simulink library "EnergyLimiterBtc"  (R2022b)
settings: Solver=VariableStepAuto  StartTime=0.0  StopTime=10.0  RelTol=1e-3
undefined symbols (not defined in the file or in its folder): magnitude
libraries: StateVar x5, AudioStats x1, FeaturePath x1, HandyTextFile x1, RTC x1
settings Model: Creator=kl13806  LastModifiedBy=kl13806
settings SolverCC: AlgebraicLoopSolver=TrustRegion
settings DebuggingCC: UnconnectedInputMsg=warning  UnconnectedOutputMsg=warning  UnconnectedLineMsg=warning  SFMachineParentedDataDiag=warning
settings ModelReferenceCC: EnableRefExpFcnMdlSchedulingChecks=on
settings RTWCC: DLArmComputeVersion=19.05

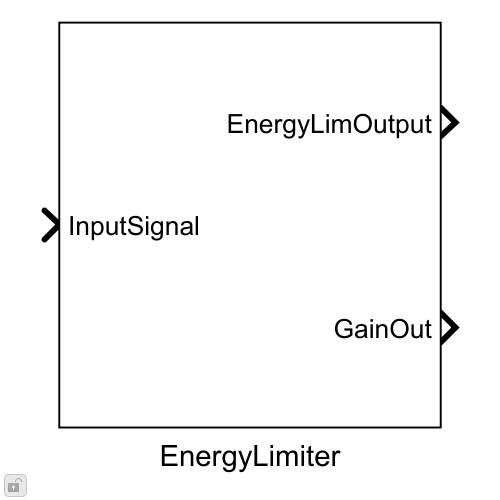
[thumbnail: Simulink's stored preview of the top-level diagram]
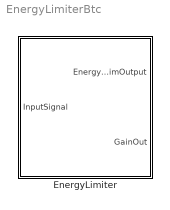
== system EnergyLimiterBtc ==
  EnergyLimiter : Subsystem  mask(Blocklib EnergyLimiter){Config=[], FeatureName=EnergyLimiterSubsystem}
      mask prompts: Config "EnergyLimiterConfig"; FeatureName "Feature path name:"
      mask help:
      | This block is used for reducing the gain of an audio signal based upon the crest factor of that signal. Such an algorithm is required for the new generations of amplifiers that have many output channels.
      |
      | Note:Please refer and click on Help tab to get details on configuration parameters
      mask init:
      | blkh=gcbh;
      | Config=BTConfig.Assert(blkh,Config);
      | 
      | Config.Validate();
      | BTConfig.InitSetFeatureIfPresent(blkh,'FeatureName');
      mask Help:
      | Configuration Parameters:
      | 
      |   GainChangeStepIndB
      |                         : Step in dB that gain should be changed by each time signal
      |                           crosses energy threshold. This number should be >= 0.
      | 
      |   GainIncreaseDurationInSeconds
      |                         : Duration that a gain increase should be applied before it
      |                           can be updated. This number should be > 0.
      | 
      |   GainDecreaseDurationInSeconds
      |                         : Duration that a gain decrease should be applied before it
      |                           can be updated. This number should be > 0.
      | 
      |   MaxEnergyLevelIndB
      |                         : Max energy level in dB for each channel above which gain
      |                           energy reduction should kick in. This number should be <= 0
      | 
      |   MaxChannels : Maximum number of channels that may be above energy level
      |                           threshold before gain reduction kicks in.
      |                           This number should be between 0 and numIn (inclusive).
      | 
      |   MaxGainReductionIndB
      |                         : Max gain reduction that should be done.
      |                           This number should be >= 0
      | 
      |   EnergyMeasurementTimeConstantInSeconds
      |                         : Time interval for averaging measured energy (in seconds).
      | 
      |   EnergyAdjustmentFactorIndB
      |                         : A Multiplier factor to adjust EBL threshold based on platform.
      |                           This number should be > 0.
      mask Callback Config: BTConfig.CallbackHideIfPresent(gcbh,{'FeatureName'});
      mask TypeOptions FeatureName: FeaturePath/FeatureName

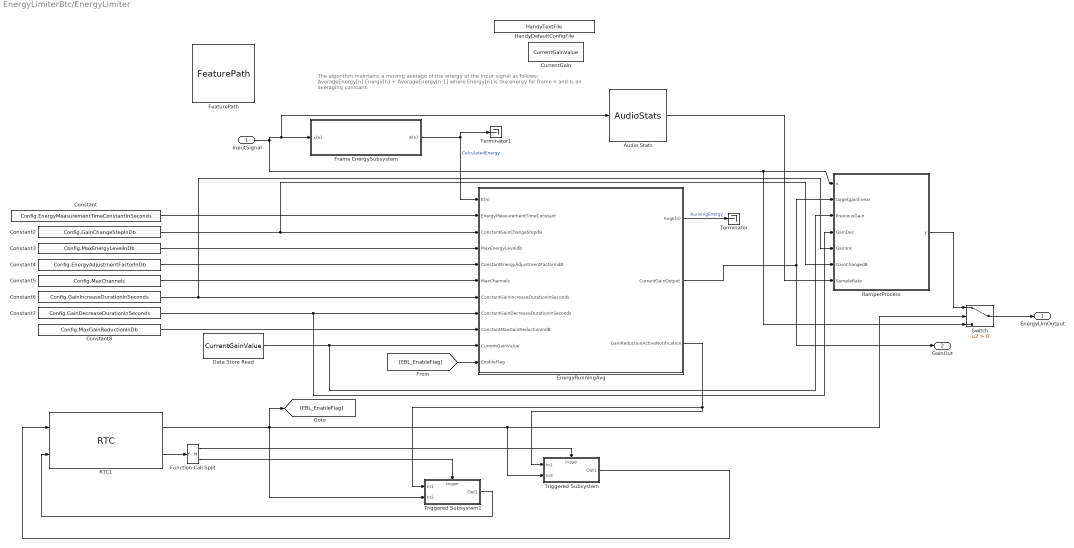
== system EnergyLimiterBtc/EnergyLimiter ==
  note: The algorithm maintains a moving average of the energy of the input signal as follows:
      | AverageEnergy[n] Energy[n] + AverageEnergy[n-1]
      | where Energy[n] is the energy for frame n and is an averaging constant.
  InputSignal : Inport
  Audio Stats : AudioStats/AudioStats  DoSampleRate=on  TypeSampleRate=Inherit: auto  DoCallRate=off  TypeCallRate=Inherit: auto  DoFrameSize=off  TypeFrameSize=Inherit: auto  DoChannelCount=off  TypeChannelCount=Inherit: auto  DoTaskRateFactor=off  TypeTaskRateFactor=Inherit: auto  MacroNameRoot=AUDIO  MacroNameRootEval='AUDIO'  IsMacroNameEval=off  MacroSampleRate=off  MacroCallRate=off  MacroFrameSize=off  MacroChannelCount=off  MacroTaskRateFactor=off  MacroTaskId=off  ValidateSampleRate=off  ValueSampleRate=[]  ValidateCallRate=off  ValueCallRate=[]  ValidateFrameSize=off  ValueFrameSize=[]  ValidateChannelCount=off  ValueChannelCount=[]  ValidateTaskRateFactor=off  ValueTaskRateFactor=[]
  Constant : Constant  Value=Config.EnergyMeasurementTimeConstantInSeconds
  Constant2 : Constant  Value=Config.GainChangeStepInDb
  Constant3 : Constant  Value=Config.MaxEnergyLevelInDb
  Constant4 : Constant  Value=Config.EnergyAdjustmentFactorInDb
  Constant5 : Constant  Value=Config.MaxChannels
  Constant6 : Constant  Value=Config.GainIncreaseDurationInSeconds
  Constant7 : Constant  Value=Config.GainDecreaseDurationInSeconds
  Constant8 : Constant  Value=Config.MaxGainReductionInDb
  CurrentGain : DataStoreMemory  DataStoreName=CurrentGainValue  InitialValue=Config.CurrentGainVal  ShowAdditionalParam=off  OutDataTypeStr=single
  Data Store Read : DataStoreRead  DataStoreName=CurrentGainValue  IndexOptions=Index vector (dialog)  Indices=1  OutputSizes=1
  "EnergyRunningAvg " : Subsystem
  FeaturePath : FeaturePath/FeaturePath  FeatureName=EnergyLimiterSubsystem  IsGroup=off  GroupNumber=-1  IsModule=off  TriggerInit=[680 174 795 281]
  Frame EnergySubsystem : Subsystem
  Function-Call Split : FunctionCallSplit  IconShape=distinctive  NumOutputPorts=2  OutputPortLayout=default
  HandyDefaultConfigFile : HandyTextFile/HandyTextFile  TemplateSource=Config  FileSuffix=Init  OpenDialogOnLoad=off  UseThisBlockName=off  TheDefaultText=|  ShowInLibBrowser=on
      | % $(FILENAME) Setup model parameters for each "Init" callback (e.g. update diagram)
      | sample_rate_in_hertz = 44100;
      | frame_size = 32;
      | sysin_channel_count = 2;
  RTC1 : RTC/RTC  REQ_Priority=RTC_Mask.NormalPriority  RequestAtInit=off  EnableRequest=off  REQElemName1=EnableGainLimiter  REQElemType1=uint32  REQElemWidth1=1  REQElemInitial1=[]  REQElemType2=uint32  REQElemWidth2=1  REQElemInitial2=[]  REQElemType3=uint32  REQElemWidth3=1  REQElemInitial3=[]  REQElemType4=uint32  REQElemWidth4=1  REQElemInitial4=[]  REQElemType5=uint32  REQElemWidth5=1  REQElemInitial5=[]  REQElemType6=uint32  REQElemWidth6=1  REQElemInitial6=[]  REQElemType7=uint32  REQElemWidth7=1  REQElemInitial7=[]  REQElemType8=uint32  REQElemWidth8=1  REQElemInitial8=[]  REQElemType9=uint32  REQElemWidth9=1  REQElemInitial9=[]  REQElemType10=uint32  REQElemWidth10=1  REQElemInitial10=[]  EnableResponse=on  EnableRSP_StatusIn=off  RSPElemType1=uint32  RSPElemWidth1=1  RSPElemType2=uint32  RSPElemWidth2=1  RSPElemType3=uint32  RSPElemWidth3=1  RSPElemType4=uint32  RSPElemWidth4=1  RSPElemType5=uint32  RSPElemWidth5=1  RSPElemType6=uint32  RSPElemWidth6=1  RSPElemType7=uint32  RSPElemWidth7=1  RSPElemType8=uint32  RSPElemWidth8=1  RSPElemType9=uint32  RSPElemWidth9=1  RSPElemType10=uint32  RSPElemWidth10=1  EnableNotification=on  EnableNTF_PrepTrig=off  NTFElemName1=ELNotification  NTFElemType1=uint32  NTFElemWidth1=1  NTFElemType2=uint32  NTFElemWidth2=1  NTFElemType3=uint32  NTFElemWidth3=1  NTFElemType4=uint32  NTFElemWidth4=1  NTFElemType5=uint32  NTFElemWidth5=1  NTFElemType6=uint32  NTFElemWidth6=1  NTFElemType7=uint32  NTFElemWidth7=1  NTFElemType8=uint32  NTFElemWidth8=1  NTFElemType9=uint32  NTFElemWidth9=1  NTFElemType10=uint32  NTFElemWidth10=1  MaskMessageName=EnableLimiter
  RamperProcess : MATLAB Function  TreatAsAtomicUnit=on
  Switch : Switch  Criteria=u2 > Threshold  SaturateOnIntegerOverflow=off  InputSameDT=off
  Terminator : Terminator
  Terminator1 : Terminator
  Triggered Subsystem : Subsystem  TreatAsAtomicUnit=on
  Triggered Subsystem1 : Subsystem  TreatAsAtomicUnit=on
  EnergyLimOutput : Outport  VectorParamsAs1DForOutWhenUnconnected=off
  GainOut : Outport  Port=2
  wires:
  Triggered Subsystem1/1(Out1) -> RTC1/2
  RTC1/2 -> Function-Call Split/1
  "EnergyRunningAvg "/1(AvgE(n)) -> Terminator/1  "RunningEnergy"
  Function-Call Split/2 -> Triggered Subsystem1/Trigger
  Constant2/1 -> RamperProcess/6(GainChangedB), "EnergyRunningAvg "/3(ConstantGainChangeStepdB)
  RamperProcess/1(y) -> Switch/1
  Function-Call Split/1 -> Triggered Subsystem/Trigger
  Triggered Subsystem/1(Out1) -> RTC1/1
  Constant6/1 -> "EnergyRunningAvg "/7(ConstantGainIncreaseDurationInSeconds), RamperProcess/5(GainInc)
  Constant/1 -> "EnergyRunningAvg "/2(EnergyMeasurementTimeConstant)
  Constant8/1 -> "EnergyRunningAvg "/9(ConstantMaxGainReductionIndB)
  InputSignal/1 -> Audio Stats/1, Frame EnergySubsystem/1(x(n)), Switch/3, RamperProcess/1(x)
  "EnergyRunningAvg "/2(CurrentGainOutput) -> GainOut/1, RamperProcess/2(targetgainlinear)
  Audio Stats/1 -> RamperProcess/7(SampleRate)
  Constant7/1 -> RamperProcess/4(GainDec), "EnergyRunningAvg "/8(ConstantGainDecreaseDurationInSeconds)
  Constant5/1 -> "EnergyRunningAvg "/6(MaxChannels)
  Constant3/1 -> "EnergyRunningAvg "/4(MaxEnergyLeveldb)
  Constant4/1 -> "EnergyRunningAvg "/5(ConstantEnergyAdjustmentFactorIndB)
  Switch/1 -> EnergyLimOutput/1
  RTC1/1 -> [EBL_EnableFlag], Triggered Subsystem1/2(In2), Triggered Subsystem/2(In3), Switch/2
  Frame EnergySubsystem/1(E(n)) -> "EnergyRunningAvg "/1(E(n)), Terminator1/1  "CalculatedEnergy"
  "EnergyRunningAvg "/3(GainReductionActiveNotification) -> Triggered Subsystem1/1(In1), Triggered Subsystem/1(In1)
  Data Store Read/1 -> "EnergyRunningAvg "/10(CurrentGainValue), RamperProcess/3(PreviousGain)
  [EBL_EnableFlag] -> "EnergyRunningAvg "/11(EnableFlag)

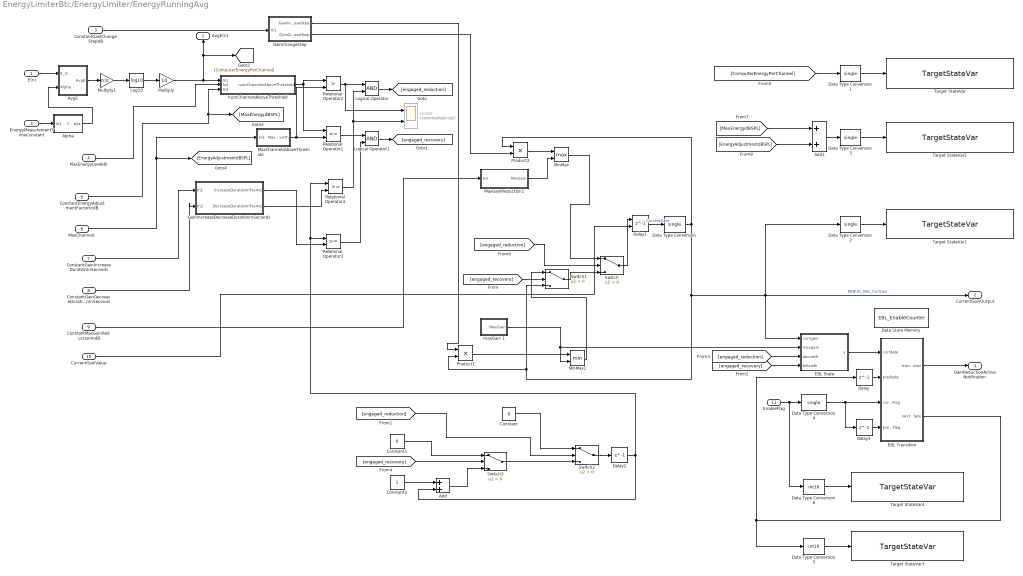
== system EnergyLimiterBtc/EnergyLimiter/EnergyRunningAvg  ==
  E(n) : Inport
  EnergyMeasurementTimeConstant : Inport  Port=2
  ConstantGainChangeStepdB : Inport  Port=3
  MaxEnergyLeveldb : Inport  Port=4
  ConstantEnergyAdjustmentFactorIndB : Inport  Port=5
  MaxChannels : Inport  Port=6
  ConstantGainIncreaseDurationInSeconds : Inport  Port=7
  ConstantGainDecreaseDurationInSeconds : Inport  Port=8
  ConstantMaxGainReductionIndB : Inport  Port=9
  CurrentGainValue : Inport  Port=10
  EnableFlag : Inport  Port=11
  Add : Sum
  Add1 : Sum
  Alpha : Subsystem
  AvgE : Subsystem
  Constant : Constant  Value=0  OutDataTypeStr=single
  Constant1 : Constant  Value=0  OutDataTypeStr=single
  Constant2 : Constant  OutDataTypeStr=single
  Data Store Memory : DataStoreMemory  DataStoreName=EBL_EnableCounter  ReadBeforeWriteMsg=warning  WriteAfterWriteMsg=warning  WriteAfterReadMsg=warning  ShowAdditionalParam=off  OutDataTypeStr=int16
  Data Type Conversion{,1..4} (5 alike) : DataTypeConversion  OutDataTypeStr=single  SaturateOnIntegerOverflow=off  RndMeth=Floor
  Data Type Conversion5 : DataTypeConversion  OutDataTypeStr=int16  SaturateOnIntegerOverflow=off  RndMeth=Floor
  Data Type Conversion6 : DataTypeConversion  OutDataTypeStr=int16  SaturateOnIntegerOverflow=off  RndMeth=Floor
  Delay : Delay  DelayLength=1
  Delay1 : Delay  DelayLength=1  InitialConditionSource=Input port
      settings: InputPortMap=u0,p4
  Delay2 : Delay  DelayLength=1  InitialCondition=1
  Delay3 : Delay  DelayLength=1
  EBL State : MATLAB Function  TreatAsAtomicUnit=on
  EBL Transition : MATLAB Function  TreatAsAtomicUnit=on
  GainChangeStep : Subsystem
  GainIncreaseDecreaseDurationInSeconds : Subsystem
  Log10 : Math  Operator=log10
  Logical Operator : Logic  AllPortsSameDT=off  OutDataTypeStr=boolean
  Logical Operator1 : Logic  AllPortsSameDT=off  OutDataTypeStr=boolean
  MaxChannelsAboveThreshold : Subsystem
  MaxGainReduction1 : Subsystem
  MinMax : MinMax  Function=max  Inputs=2  OutDataTypeStr=single
  MinMax1 : MinMax  Inputs=2  OutDataTypeStr=single
  Multiply : Gain  Gain=10
  Multiply1 : Gain  Gain=2/32
  Product1 : Product  OutDataTypeStr=single
  Product2 : Product
  Relational Operator1 : RelationalOperator  Operator=<=  OutDataTypeStr=boolean  RndMeth=Simplest  InputSameDT=off
  Relational Operator2 : RelationalOperator  Operator=>  OutDataTypeStr=boolean  RndMeth=Simplest  InputSameDT=off
  Relational Operator3 : RelationalOperator  OutDataTypeStr=boolean  RndMeth=Simplest  InputSameDT=off
  Relational Operator4 : RelationalOperator  OutDataTypeStr=boolean  RndMeth=Simplest  InputSameDT=off
  Scope : Scope  Commented=on  NumInputPorts=2
  Switch{,1..3} (4 alike) : Switch  Criteria=u2 > Threshold  SaturateOnIntegerOverflow=off  InputSameDT=off
  Target StateVar : StateVar/TargetStateVar  TriggerInit=[1755 218 2035 282]  TspName=ComputedEnergy  StateName=ComputedEnergy  UseSameName=on  IfdefMacro=[]
  Target StateVar1 : StateVar/TargetStateVar  TriggerInit=[1755 548 2035 612]  TspName=CurGain  StateName=CurGain  UseSameName=on  IfdefMacro=[]
  Target StateVar2 : StateVar/TargetStateVar  TriggerInit=[1755 358 2035 422]  TspName=EnergyThreshold  StateName=EnergyThreshold  UseSameName=on  IfdefMacro=[]
  Target StateVar3 : StateVar/TargetStateVar  TriggerInit=[1680 1253 1925 1317]  TspName=CurState  StateName=CurState  UseSameName=on  IfdefMacro=[]
  Target StateVar4 : StateVar/TargetStateVar  TriggerInit=[1680 1123 1925 1187]  TspName=EnableFlag  StateName=EnableFlag  UseSameName=on  IfdefMacro=[]
  maxGain 1 : Subsystem
  numChannelsAboveThreshold : Subsystem
  AvgE(n) : Outport  VectorParamsAs1DForOutWhenUnconnected=off
  CurrentGainOutput : Outport  Port=2  VectorParamsAs1DForOutWhenUnconnected=off
  GainReductionActiveNotification : Outport  Port=3  VectorParamsAs1DForOutWhenUnconnected=off
  wires:
  EBL Transition/2(nextState) -> Data Type Conversion5/1, Delay/1
  Add/1 -> Switch3/3
  Constant2/1 -> Add/1
  CurrentGainValue/1 -> Delay1/2
  ConstantMaxGainReductionIndB/1 -> MaxGainReduction1/1(In1)
  ConstantGainDecreaseDurationInSeconds/1 -> GainIncreaseDecreaseDurationInSeconds/2(In2)
  ConstantGainIncreaseDurationInSeconds/1 -> GainIncreaseDecreaseDurationInSeconds/1(In1)
  MaxChannels/1 -> [EnergyAdjustmentdBSPL], MaxChannelsAboveThreshold/1(In1)
  ConstantEnergyAdjustmentFactorIndB/1 -> [MaxEnergydBSPL], numChannelsAboveThreshold/3(In3)
  MaxEnergyLeveldb/1 -> numChannelsAboveThreshold/2(In2)
  ConstantGainChangeStepdB/1 -> GainChangeStep/1(In1)
  EnergyMeasurementTimeConstant/1 -> Alpha/1(In1)
  Delay2/1 -> Relational Operator4/1, Relational Operator3/1, Add/2
  Switch3/1 -> Switch2/3
  Constant/1 -> Switch2/1
  [engaged_recovery] -> Switch3/2
  [engaged_reduction] -> Switch2/2
  Switch/1 -> Delay1/1
  Product1/1 -> MinMax1/1
  Delay1/1 -> Data Type Conversion/1  "CurrentGain"
  Switch1/1 -> Switch/3
  MinMax1/1 -> Switch1/1
  [engaged_recovery] -> Switch1/2
  [engaged_reduction] -> Switch/2
  Switch2/1 -> Delay2/1
  MinMax/1 -> Switch/1
  maxGain 1/1(MaxGain) -> MinMax1/2, EBL State/2(maxgain)
  GainChangeStep/1(GainIncreaseStep) -> Product1/1
  MaxGainReduction1/1(MinGain) -> MinMax/2
  GainChangeStep/2(GainDecreaseStep) -> Product2/2
  Product2/1 -> MinMax/1
  Logical Operator/1 -> [engaged_reduction]
  Logical Operator1/1 -> [engaged_recovery]
  Relational Operator3/1 -> Logical Operator1/2
  Relational Operator1/1 -> Logical Operator1/1
  Relational Operator4/1 -> Logical Operator/2, Scope/2
  Relational Operator2/1 -> Logical Operator/1, Scope/1
  GainIncreaseDecreaseDurationInSeconds/2(DecreaseDurationInFrame) -> Relational Operator4/2
  GainIncreaseDecreaseDurationInSeconds/1(IncreaseDurationInFrame) -> Relational Operator3/2
  MaxChannelsAboveThreshold/1(MaxChAboveTh) -> Relational Operator1/2, Relational Operator2/2
  numChannelsAboveThreshold/1(numChannelsAboveThreshold) -> Relational Operator1/1, Relational Operator2/1
  Alpha/1(CoffAlpha) -> AvgE/2(Alpha)
  E(n)/1 -> AvgE/1(E_In)
  Data Type Conversion/1 -> Data Type Conversion2/1, EBL State/1(currgain), CurrentGainOutput/1, Switch1/3, Product1/2, Product2/1  "DEBUG_EBL_CurGain"
  Multiply/1 -> [ComputerEnergyPerChannel], AvgE(n)/1, numChannelsAboveThreshold/1(In1)
  Log10/1 -> Multiply/1
  AvgE/1(AvgE) -> Multiply1/1
  Multiply1/1 -> Log10/1
  [engaged_recovery] -> EBL State/4(belowth)
  [engaged_reduction] -> EBL State/3(aboveth)
  EBL Transition/1(transition) -> GainReductionActiveNotification/1
  Delay/1 -> EBL Transition/2(preState)
  EBL State/1(y) -> EBL Transition/1(curState)
  Constant1/1 -> Switch3/1
  Data Type Conversion1/1 -> Target StateVar/1
  [ComputerEnergyPerChannel] -> Data Type Conversion1/1
  Data Type Conversion2/1 -> Target StateVar1/1
  Add1/1 -> Data Type Conversion3/1
  [MaxEnergydBSPL] -> Add1/1
  [EnergyAdjustmentdBSPL] -> Add1/2
  Data Type Conversion3/1 -> Target StateVar2/1
  EnableFlag/1 -> Data Type Conversion6/1, Data Type Conversion4/1
  Delay3/1 -> EBL Transition/4(preEnableFlag)
  Data Type Conversion4/1 -> EBL Transition/3(curEnableFlag), Delay3/1
  Data Type Conversion5/1 -> Target StateVar3/1
  Data Type Conversion6/1 -> Target StateVar4/1

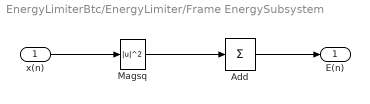
== system EnergyLimiterBtc/EnergyLimiter/Frame EnergySubsystem ==
  x(n) : Inport
  Add : Sum  Inputs=+  CollapseMode=Specified dimension
  Magsq : Math  Operator=magnitude^2  SignedPower=on
  E(n) : Outport  VectorParamsAs1DForOutWhenUnconnected=off
  wires:
  x(n)/1 -> Magsq/1
  Magsq/1 -> Add/1
  Add/1 -> E(n)/1

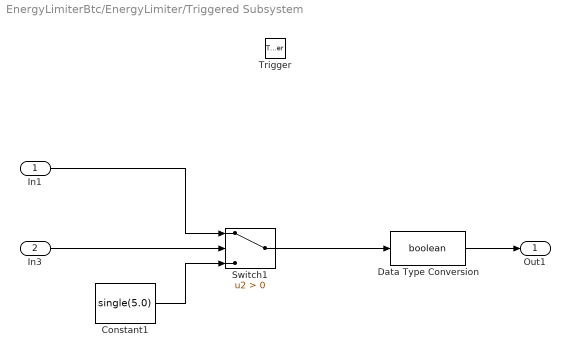
== system EnergyLimiterBtc/EnergyLimiter/Triggered Subsystem ==
  In1 : Inport
  In3 : Inport  Port=2
  Trigger : TriggerPort  TriggerType=function-call  VariantControl=Variant
  Constant1 : Constant  Value=single(5.0)  OutDataTypeStr=single
  Data Type Conversion : DataTypeConversion  OutDataTypeStr=boolean  SaturateOnIntegerOverflow=off  RndMeth=Floor
  Switch1 : Switch  Criteria=u2 > Threshold  SaturateOnIntegerOverflow=off  InputSameDT=off
  Out1 : Outport
  wires:
  In1/1 -> Switch1/1
  Data Type Conversion/1 -> Out1/1
  Constant1/1 -> Switch1/3
  Switch1/1 -> Data Type Conversion/1
  In3/1 -> Switch1/2

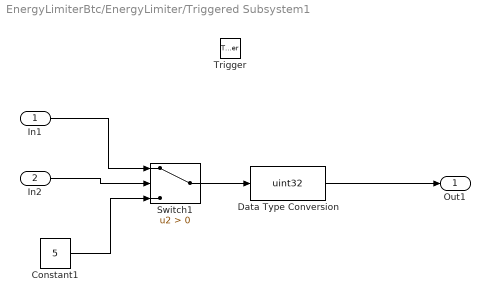
== system EnergyLimiterBtc/EnergyLimiter/Triggered Subsystem1 ==
  In1 : Inport
  In2 : Inport  Port=2
  Trigger : TriggerPort  TriggerType=function-call  VariantControl=Variant
  Constant1 : Constant  Value=5  OutDataTypeStr=single
  Data Type Conversion : DataTypeConversion  OutDataTypeStr=uint32  SaturateOnIntegerOverflow=off  RndMeth=Floor
  Switch1 : Switch  Criteria=u2 > Threshold  SaturateOnIntegerOverflow=off  InputSameDT=off
  Out1 : Outport  VectorParamsAs1DForOutWhenUnconnected=off
  wires:
  In1/1 -> Switch1/1
  Data Type Conversion/1 -> Out1/1
  Constant1/1 -> Switch1/3
  In2/1 -> Switch1/2
  Switch1/1 -> Data Type Conversion/1

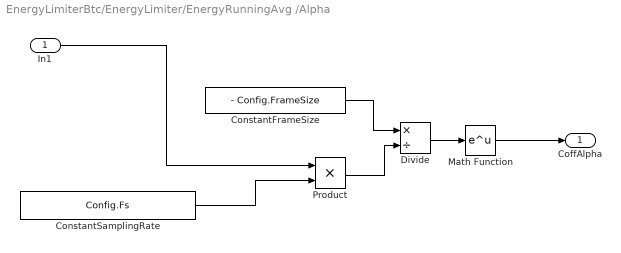
== system EnergyLimiterBtc/EnergyLimiter/EnergyRunningAvg /Alpha ==
  In1 : Inport
  ConstantFrameSize : Constant  Value=- Config.FrameSize  OutDataTypeStr=single
  ConstantSamplingRate : Constant  Value=Config.Fs  OutDataTypeStr=single
  Divide : Product  Inputs=*/
  Math Function : Math  SignedPower=on
  Product : Product
  CoffAlpha : Outport  VectorParamsAs1DForOutWhenUnconnected=off
  wires:
  In1/1 -> Product/1
  Product/1 -> Divide/2
  Math Function/1 -> CoffAlpha/1
  ConstantSamplingRate/1 -> Product/2
  Divide/1 -> Math Function/1
  ConstantFrameSize/1 -> Divide/1

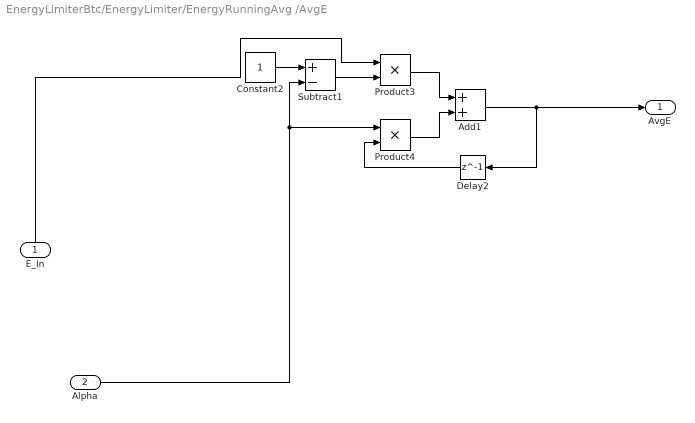
== system EnergyLimiterBtc/EnergyLimiter/EnergyRunningAvg /AvgE ==
  E_In : Inport
  Alpha : Inport  Port=2
  Add1 : Sum
  Constant2 : Constant  OutDataTypeStr=single
  Delay2 : Delay  DelayLength=1  InitialCondition=0
  Product3 : Product
  Product4 : Product
  Subtract1 : Sum  Inputs=+-
  AvgE : Outport  VectorParamsAs1DForOutWhenUnconnected=off
  wires:
  Alpha/1 -> Product4/1, Subtract1/2
  Product3/1 -> Add1/1
  Constant2/1 -> Subtract1/1
  E_In/1 -> Product3/1
  Product4/1 -> Add1/2
  Delay2/1 -> Product4/2
  Add1/1 -> Delay2/1, AvgE/1
  Subtract1/1 -> Product3/2

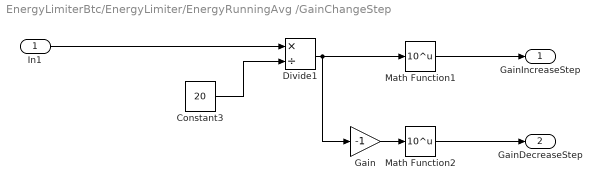
== system EnergyLimiterBtc/EnergyLimiter/EnergyRunningAvg /GainChangeStep ==
  In1 : Inport
  Constant3 : Constant  Value=20  OutDataTypeStr=single
  Divide1 : Product  Inputs=*/
  Gain : Gain  Gain=-1
  Math Function1 : Math  Operator=10^u  SignedPower=on
  Math Function2 : Math  Operator=10^u  SignedPower=on
  GainIncreaseStep : Outport  VectorParamsAs1DForOutWhenUnconnected=off
  GainDecreaseStep : Outport  Port=2  VectorParamsAs1DForOutWhenUnconnected=off
  wires:
  Math Function2/1 -> GainDecreaseStep/1
  Math Function1/1 -> GainIncreaseStep/1
  In1/1 -> Divide1/1
  Divide1/1 -> Math Function1/1, Gain/1
  Gain/1 -> Math Function2/1
  Constant3/1 -> Divide1/2

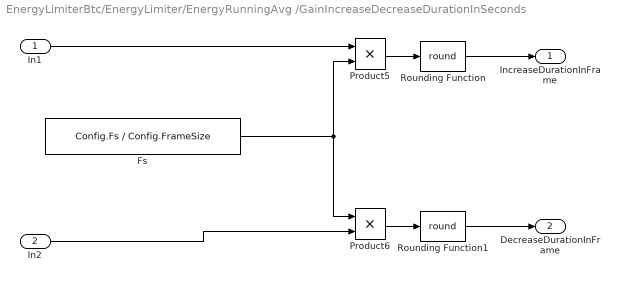
== system EnergyLimiterBtc/EnergyLimiter/EnergyRunningAvg /GainIncreaseDecreaseDurationInSeconds ==
  In1 : Inport
  In2 : Inport  Port=2
  Fs : Constant  Value=Config.Fs / Config.FrameSize  OutDataTypeStr=single
  Product5 : Product
  Product6 : Product
  Rounding Function : Rounding  Operator=round
  Rounding Function1 : Rounding  Operator=round
  IncreaseDurationInFrame : Outport  VectorParamsAs1DForOutWhenUnconnected=off
  DecreaseDurationInFrame : Outport  Port=2  VectorParamsAs1DForOutWhenUnconnected=off
  wires:
  Fs/1 -> Product5/2, Product6/1
  In1/1 -> Product5/1
  Product6/1 -> Rounding Function1/1
  Product5/1 -> Rounding Function/1
  In2/1 -> Product6/2
  Rounding Function/1 -> IncreaseDurationInFrame/1
  Rounding Function1/1 -> DecreaseDurationInFrame/1

== system EnergyLimiterBtc/EnergyLimiter/EnergyRunningAvg /MaxChannelsAboveThreshold ==
  In1 : Inport
  Rounding Function : Rounding  Operator=round
  MaxChAboveTh : Outport  VectorParamsAs1DForOutWhenUnconnected=off
  wires:
  Rounding Function/1 -> MaxChAboveTh/1
  In1/1 -> Rounding Function/1

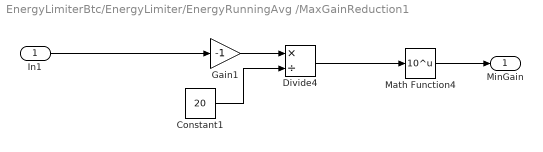
== system EnergyLimiterBtc/EnergyLimiter/EnergyRunningAvg /MaxGainReduction1 ==
  In1 : Inport
  Constant1 : Constant  Value=20  OutDataTypeStr=single
  Divide4 : Product  Inputs=*/
  Gain1 : Gain  Gain=-1
  Math Function4 : Math  Operator=10^u  SignedPower=on
  MinGain : Outport  VectorParamsAs1DForOutWhenUnconnected=off
  wires:
  Math Function4/1 -> MinGain/1
  Divide4/1 -> Math Function4/1
  Constant1/1 -> Divide4/2
  In1/1 -> Gain1/1
  Gain1/1 -> Divide4/1

== system EnergyLimiterBtc/EnergyLimiter/EnergyRunningAvg /maxGain 1 ==
  Constant1 : Constant  OutDataTypeStr=single
  MaxGain : Outport  VectorParamsAs1DForOutWhenUnconnected=off
  wires:
  Constant1/1 -> MaxGain/1

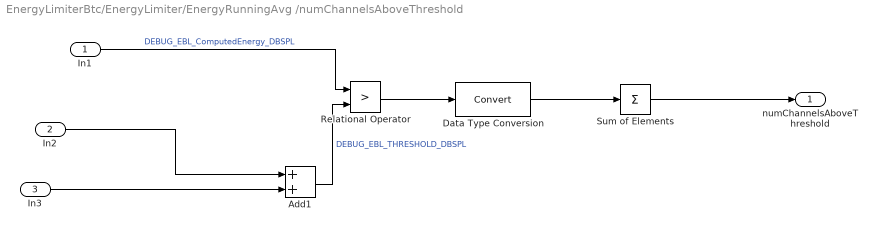
== system EnergyLimiterBtc/EnergyLimiter/EnergyRunningAvg /numChannelsAboveThreshold ==
  In1 : Inport
  In2 : Inport  Port=2
  In3 : Inport  Port=3
  Add1 : Sum
  Data Type Conversion : DataTypeConversion  SaturateOnIntegerOverflow=off  RndMeth=Floor
  Relational Operator : RelationalOperator  Operator=>  OutDataTypeStr=boolean  RndMeth=Simplest  InputSameDT=off
  Sum of Elements : Sum  Inputs=+
  numChannelsAboveThreshold : Outport  VectorParamsAs1DForOutWhenUnconnected=off
  wires:
  In1/1 -> Relational Operator/1  "DEBUG_EBL_ComputedEnergy_DBSPL"
  Sum of Elements/1 -> numChannelsAboveThreshold/1
  In3/1 -> Add1/2
  Add1/1 -> Relational Operator/2  "DEBUG_EBL_THRESHOLD_DBSPL"
  In2/1 -> Add1/1
  Relational Operator/1 -> Data Type Conversion/1
  Data Type Conversion/1 -> Sum of Elements/1

== matlab function EnergyLimiterBtc/EnergyLimiter/EnergyRunningAvg /EBL Transition ==
  data: curState input; transition output; preState input; curEnableFlag input single; nextState output single; preEnableFlag input single
function [transition, nextState] = fcn(curState,preState,curEnableFlag,preEnableFlag)
%
% Calculate EBL states
%
% Calculate next state and transition from previous state, current state, previous enable
% flag, and current enable flag
%

persistent EBL_EnableCounter;
if isempty(EBL_EnableCounter) EBL_EnableCounter=int16(0); end

% List of all EBL states and transitions
EBL_EnableFlag_False         = single(0.0);
EBL_EnableFlag_True          = single(1.0);
EBL_StateNoUpdate            = single(0.0); 
EBL_StateAttackInProgress    = single(1.0); 
EBL_StateRecoveryInProgress  = single(2.0); 
EBL_StateDisengaged          = single(3.0); 
EBL_TransitionNoChange       = single(0.0); 
EBL_TransitionAttackStart    = single(1.0); 
EBL_TransitionRecoverDone    = single(2.0); 

% First, check if the enable flag is updated
if(preState==EBL_StateAttackInProgress     && ...
        curEnableFlag==EBL_EnableFlag_True && ...
        preEnableFlag==EBL_EnableFlag_False)
    EBL_EnableCounter = EBL_EnableCounter+1;
    % EBL enabled while attack in progress
    transition=EBL_TransitionAttackStart;
    if(curState == EBL_StateNoUpdate) 
        nextState=preState;
    else
        nextState=curState;
    end    
    return;
end

% Check if the EBL state is updated
if(curState == EBL_StateNoUpdate)  
    transition=EBL_TransitionNoChange;
    nextState=preState;
    return;
else
    nextState=curState;
end

% Determine the transition based on EBL state
if(preState==EBL_StateDisengaged && ...
   curState==EBL_StateAttackInProgress)
    % attack begins
    transition=EBL_TransitionAttackStart;
elseif(preState==EBL_StateRecoveryInProgress && ...
       curState==EBL_StateDisengaged)
    % recovery done
    transition=EBL_TransitionRecoverDone;
else
    transition=EBL_TransitionNoChange;
end

== matlab function EnergyLimiterBtc/EnergyLimiter/EnergyRunningAvg /EBL State ==
  data: currgain input; y output; maxgain input; aboveth input; belowth input
function y = fcn(currgain,maxgain,aboveth,belowth)
%
% Return gain notifications based on current gain and thresholds
%

ELNotification = single(0);
if((currgain<maxgain))
    if(aboveth)
    %% Gain reduction when energy limiter active
       ELNotification = single(1.0);
    end
    %if((currgain==mingain))
    if(belowth)
        %% Increased gain notification when energy limiter active
        ELNotification= single(2.0);
    end
elseif(currgain== maxgain)
    %% No Gain reduction when energy limiter active
    ELNotification= single(3.0);
else
    ELNotification= single(4.0);
end

y = single(ELNotification);

== matlab function EnergyLimiterBtc/EnergyLimiter/RamperProcess ==
  data: x input; y output; targetgainlinear input; PreviousGain input; GainDec input; GainInc input; GainChangedB input; SampleRate input
function y = fcn(x,targetgainlinear,PreviousGain,GainDec,GainInc,GainChangedB,SampleRate)
M = 1; % for matlab 1 based indexing
nf = single(size(x,1)); % get the frame size. DO NOT USE length() since it may
y = single(zeros(size(x)));
% more channels than samples per frame.
%Defines for status
RAMP_IDLE        = 0; RAMPING_UP       = 1; RAMPING_DOWN     = -1;

numChs = single(size(x,2)); numRampers = 1;
% Configure the rgain block to have an attack (or decay) rate that
% is twice as fast as the ratio of GainChangeStepIndB to
% GainIncreaseDurationInSeconds (or
% GainDecreaseDurationInSeconds). That way, the rgain block will
% have settled to the target value before a new gain change occurs.
rampUpRates_dBPerSec= (2*GainChangedB/GainInc); rampDownRates_dBPerSec=(-2*GainChangedB/GainDec);
frameSize=nf; Fs=SampleRate; lpfTau=frameSize/Fs; snapThresh=single(1e-5); mindB=single(-100.0);


upCoeff       = undb20(rampUpRates_dBPerSec/Fs); upCoeffN  = upCoeff .^ frameSize;
downCoeff     = undb20(-abs(rampDownRates_dBPerSec)/Fs); downCoeffN  = downCoeff .^ frameSize;
lpfCoeff      = single(exp(-1./(lpfTau.*Fs))); minGain = undb20(mindB);
targetCoeffSet =single(zeros(numRampers,1)); activeCoeffSet =single(zeros(numRampers,1));
status = RAMP_IDLE; freeze=single(0.0);
targetRamper =single(zeros(numChs,1)); activeRamper=single(zeros(numChs,1));
persistent prevGain;
if(isempty(prevGain))
    prevGain=single((PreviousGain*ones(numRampers,1)));
end
targetGain=targetgainlinear;
if(targetgainlinear<1)
    %disp('done');
end
rGain=single(zeros(numRampers,1));


% simulate use of scratch buffers for ramped envelopes
scratchBufs = single(zeros(nf,numRampers)); 
% loop over rampers first
for r = 1:numRampers
    % update active set with target
   activeCoeffSet(r) = targetCoeffSet(r);
   setIdx = activeCoeffSet(r) + M;
   % get all coeffs from active set
   lpfCoeff = lpfCoeff(setIdx);
   
   gp = prevGain(r);
   if freeze
      gt = gp; 
   else
      gt = targetGain(r); 
   end
   gdiff = gt-gp;
   
    % Snap to target gain if it's close enough
    if( abs(gdiff) <= snapThresh )
      prevGain(r) = gt;
      status(r) = RAMP_IDLE;
      scratchBufs(:,r) = gt;
      continue;         % Done with this channel, continue to next channel
    end

    % Ramp up or down?
    if( gdiff>0 )
        status(r) = RAMPING_UP;

        % Check for ramp done
        temp = max(gp,minGain);  % previous gain cannot be zero for exponential ramp
        if( temp*upCoeffN(setIdx) < gt )
            % Ramp not done, so do zero-input exponential ramp
            a = upCoeff(setIdx);  b0 = single(0.0);  gp = temp;
        else
            % LPF with target gain as input
            a = lpfCoeff; b0 = 1-a;
        end
    else
        status(r) = RAMPING_DOWN;
        % Check for ramp done
        if( gp*downCoeffN(setIdx) > gt )
            % Ramp not done, so do zero-input exponential ramp
            a = downCoeff(setIdx);  b0 = single(0.0);
        else
            % LPF with target gain as input
            a = lpfCoeff;  b0 = 1-a;
        end
    end
    % Calculate gain envelope for current ramper
%     zi = a*gp;    % initial condition for filter
%     scratchBufs(:,r) = filter(b0,[1 -a],gt*ones(nf,1),zi);
    % use single() to force MATLAB to compute gain envelope in 32-bit
    % precision to match the performance of current 32-bit DSP processors
    for k = 1:nf
        %scratchBufs(k,r) = double(single(b0)*single(gt) + (single(a)*single(gp))); 
        scratchBufs(k,r) = b0*gt + a*gp;   gp = scratchBufs(k,r);
    end
    % save state
    prevGain(r) = scratchBufs(end,r);
     
end
% then apply ramped gains to channels
for ch = 1:numChs
    activeRamper(ch) = targetRamper(ch); % update active ramper with target
    if  activeRamper(ch) ~= -1
        rGain = scratchBufs(:,activeRamper(ch) + M); % get ramped envelope assigned to ch
        y(:,ch) = rGain.*x(:,ch);
    else
        y(:,ch) = 0;
    end
end
